simulink model "viet_HC_arbot_v2offset"  (R2020a)
settings: Solver=ode15s  StartTime=0.0  StopTime=15  MaxStep=.01  RelTol=1e-3  AbsTol=1e-4
InitFcn:
  | % currentFolder = pwd;
  | % parent = '../Targeting';
  | % environment = '../Environment';
  | % addpath(genpath(parent));
  | % addpath(genpath(environment));
  | 
  | startup_ARbot;
  | chute2_DataFile;
  | guard_DataFile1;
  | shelf_DataFile1;
  | bin_assembly_DataFile;
values from neighbouring files (symbols this model uses):
  base_link = which('base_link.STL')    [init_root_paths_mac.m]    (also in init_root_paths_windows.m)
  Environment = append(cwd,'/Environment')    [init_root_paths_mac.m]    (also in init_root_paths_windows.m = append(cwd,'\Environment'))
  L1 = which('L1.STL')    [init_root_paths_mac.m]    (also in init_root_paths_windows.m)
  L2 = which('L2.STL')    [init_root_paths_mac.m]    (also in init_root_paths_windows.m)
  L3 = which('L3.STL')    [init_root_paths_mac.m]    (also in init_root_paths_windows.m)
  L4 = which('L4.STL')    [init_root_paths_mac.m]    (also in init_root_paths_windows.m)
undefined symbols (not defined in the file or in its folder): belt_h, belt_l, belt_spd, belt_w, box1_dim, box2_dim, box3_dim, box4_dim, box5_dim, cube_d, deposit_joint_angle, Extr_Data_LinkHoles, floor_d, floor_l, ikSol, initial_joints, m, n, P_C, safe_via_angles, sigbuilder_block, smiData, X, Y, Z
libraries: sm_lib x145, nesl_utility x78, Contact_Forces_Lib x10, simulink x5, Parts_Lib x5, dspsrcs4 x1
(part 5 of 5)

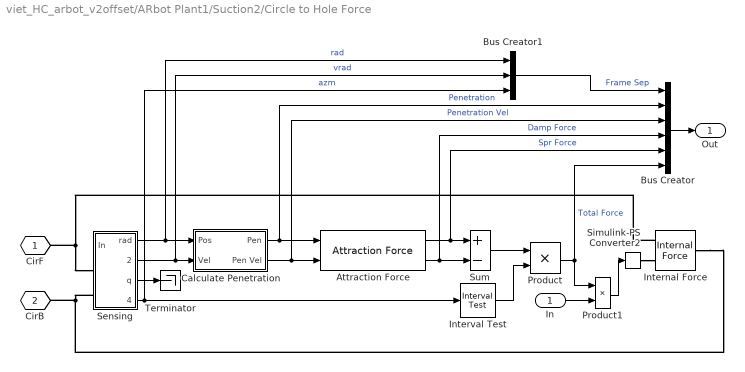
== system viet_HC_arbot_v2offset/ARbot Plant1/Suction2/Circle to Hole Force ==
  In : Inport
  Attraction Force : Contact_Forces_Lib/Other Forces/Attraction Force  k_pen=k_contact  b_penvel=b_contact  max_sep=max_frame_sep  deadzone=h_deadzone
      settings: SourceProductName=Simscape Multibody Contact Forces Library
  Bus Creator : BusCreator  Inputs=6
  Bus Creator1 : BusCreator  Inputs=3
  Calculate Penetration : Subsystem
  Internal Force : sm_lib/Forces and Torques/Internal Force
      settings: SourceProductBaseCode=MS
  Interval Test : simulink/Logic and Bit Operations/Interval Test  IntervalClosedRight=on  uplimit=active_angle(2)  IntervalClosedLeft=on  lowlimit=active_angle(1)  OutDataTypeStr=uint8
  Product : Product
  Product1 : Product
  Sensing : Subsystem
  Simulink-PS Converter2 : nesl_utility/Simulink-PS Converter  PhysicalDomain=network_engine_domain  SubClassName=ps_input  LeftPortType=input  RightPortType=output  PseudoPeriodic=off  Frequencies=[]  NoiseDistribution=none  NoiseParameters=[]  Unit=1  AffineConversion=off  FilteringAndDerivatives=zero  SimscapeFilterOrder=1  InputFilterTimeConstant=0.005  UdotUserProvided=[]
  Sum : Sum  Inputs=+-
  Terminator : Terminator
  CirF : PMIOPort  Tag=PMCPort  Side=Left
  CirB : PMIOPort  Tag=PMCPort  Port=2  Side=Right
  Out : Outport  VectorParamsAs1DForOutWhenUnconnected=off
  wires:
  Product1/1 -> Simulink-PS Converter2/1
  In/1 -> Product1/2
  Interval Test/1 -> Product/2
  Sensing/3(q) -> Terminator/1
  Sum/1 -> Product/1
  Attraction Force/1 -> Bus Creator/5, Sum/1  "Spr Force"
  Sensing/1(rad) -> Bus Creator1/1, Calculate Penetration/1(Pos)  "rad"
  Attraction Force/2 -> Bus Creator/4, Sum/2  "Damp Force"
  Sensing/2(vrad) -> Bus Creator1/2, Calculate Penetration/2(Vel)  "vrad"
  Calculate Penetration/2(Pen Vel) -> Attraction Force/2, Bus Creator/3  "Penetration Vel"
  Product/1 -> Bus Creator/6, Product1/1  "Total Force"
  Sensing/4(azm) -> Bus Creator1/3, Interval Test/1  "azm"
  Bus Creator1/1 -> Bus Creator/1  "Frame Sep"
  Calculate Penetration/1(Pen) -> Attraction Force/1, Bus Creator/2  "Penetration"
  Bus Creator/1 -> Out/1
  connections:
  Sensing/LConn2 -- Internal Force/RConn1 -- CirB/RConn1
  Internal Force/LConn1 -- Sensing/LConn1 -- CirF/RConn1
  Simulink-PS Converter2/RConn1 -- Internal Force/LConn2

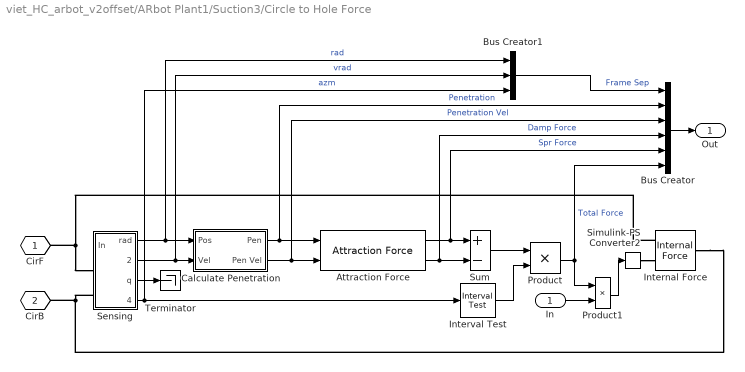
== system viet_HC_arbot_v2offset/ARbot Plant1/Suction3/Circle to Hole Force ==
  In : Inport
  Attraction Force : Contact_Forces_Lib/Other Forces/Attraction Force  k_pen=k_contact  b_penvel=b_contact  max_sep=max_frame_sep  deadzone=h_deadzone
      settings: SourceProductName=Simscape Multibody Contact Forces Library
  Bus Creator : BusCreator  Inputs=6
  Bus Creator1 : BusCreator  Inputs=3
  Calculate Penetration : Subsystem
  Internal Force : sm_lib/Forces and Torques/Internal Force
      settings: SourceProductBaseCode=MS
  Interval Test : simulink/Logic and Bit Operations/Interval Test  IntervalClosedRight=on  uplimit=active_angle(2)  IntervalClosedLeft=on  lowlimit=active_angle(1)  OutDataTypeStr=uint8
  Product : Product
  Product1 : Product
  Sensing : Subsystem
  Simulink-PS Converter2 : nesl_utility/Simulink-PS Converter  PhysicalDomain=network_engine_domain  SubClassName=ps_input  LeftPortType=input  RightPortType=output  PseudoPeriodic=off  Frequencies=[]  NoiseDistribution=none  NoiseParameters=[]  Unit=1  AffineConversion=off  FilteringAndDerivatives=zero  SimscapeFilterOrder=1  InputFilterTimeConstant=0.005  UdotUserProvided=[]
  Sum : Sum  Inputs=+-
  Terminator : Terminator
  CirF : PMIOPort  Tag=PMCPort  Side=Left
  CirB : PMIOPort  Tag=PMCPort  Port=2  Side=Right
  Out : Outport  VectorParamsAs1DForOutWhenUnconnected=off
  wires:
  Bus Creator/1 -> Out/1
  Calculate Penetration/1(Pen) -> Bus Creator/2, Attraction Force/1  "Penetration"
  Bus Creator1/1 -> Bus Creator/1  "Frame Sep"
  Sensing/4(azm) -> Interval Test/1, Bus Creator1/3  "azm"
  Product/1 -> Product1/1, Bus Creator/6  "Total Force"
  Calculate Penetration/2(Pen Vel) -> Bus Creator/3, Attraction Force/2  "Penetration Vel"
  Sensing/2(vrad) -> Calculate Penetration/2(Vel), Bus Creator1/2  "vrad"
  Attraction Force/2 -> Sum/2, Bus Creator/4  "Damp Force"
  Sensing/1(rad) -> Calculate Penetration/1(Pos), Bus Creator1/1  "rad"
  Attraction Force/1 -> Sum/1, Bus Creator/5  "Spr Force"
  Sum/1 -> Product/1
  Sensing/3(q) -> Terminator/1
  Interval Test/1 -> Product/2
  In/1 -> Product1/2
  Product1/1 -> Simulink-PS Converter2/1
  connections:
  Simulink-PS Converter2/RConn1 -- Internal Force/LConn2
  CirF/RConn1 -- Sensing/LConn1 -- Internal Force/LConn1
  CirB/RConn1 -- Internal Force/RConn1 -- Sensing/LConn2

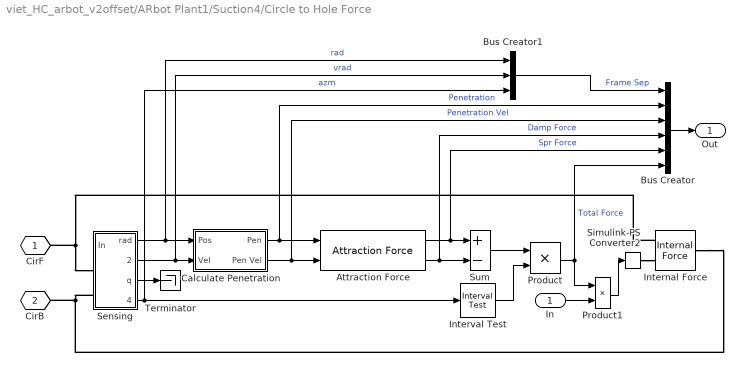
== system viet_HC_arbot_v2offset/ARbot Plant1/Suction4/Circle to Hole Force ==
  In : Inport
  Attraction Force : Contact_Forces_Lib/Other Forces/Attraction Force  k_pen=k_contact  b_penvel=b_contact  max_sep=max_frame_sep  deadzone=h_deadzone
      settings: SourceProductName=Simscape Multibody Contact Forces Library
  Bus Creator : BusCreator  Inputs=6
  Bus Creator1 : BusCreator  Inputs=3
  Calculate Penetration : Subsystem
  Internal Force : sm_lib/Forces and Torques/Internal Force
      settings: SourceProductBaseCode=MS
  Interval Test : simulink/Logic and Bit Operations/Interval Test  IntervalClosedRight=on  uplimit=active_angle(2)  IntervalClosedLeft=on  lowlimit=active_angle(1)  OutDataTypeStr=uint8
  Product : Product
  Product1 : Product
  Sensing : Subsystem
  Simulink-PS Converter2 : nesl_utility/Simulink-PS Converter  PhysicalDomain=network_engine_domain  SubClassName=ps_input  LeftPortType=input  RightPortType=output  PseudoPeriodic=off  Frequencies=[]  NoiseDistribution=none  NoiseParameters=[]  Unit=1  AffineConversion=off  FilteringAndDerivatives=zero  SimscapeFilterOrder=1  InputFilterTimeConstant=0.005  UdotUserProvided=[]
  Sum : Sum  Inputs=+-
  Terminator : Terminator
  CirF : PMIOPort  Tag=PMCPort  Side=Left
  CirB : PMIOPort  Tag=PMCPort  Port=2  Side=Right
  Out : Outport  VectorParamsAs1DForOutWhenUnconnected=off
  wires:
  Product1/1 -> Simulink-PS Converter2/1
  In/1 -> Product1/2
  Interval Test/1 -> Product/2
  Sensing/3(q) -> Terminator/1
  Sum/1 -> Product/1
  Attraction Force/1 -> Bus Creator/5, Sum/1  "Spr Force"
  Sensing/1(rad) -> Bus Creator1/1, Calculate Penetration/1(Pos)  "rad"
  Attraction Force/2 -> Bus Creator/4, Sum/2  "Damp Force"
  Sensing/2(vrad) -> Bus Creator1/2, Calculate Penetration/2(Vel)  "vrad"
  Calculate Penetration/2(Pen Vel) -> Attraction Force/2, Bus Creator/3  "Penetration Vel"
  Product/1 -> Bus Creator/6, Product1/1  "Total Force"
  Sensing/4(azm) -> Bus Creator1/3, Interval Test/1  "azm"
  Bus Creator1/1 -> Bus Creator/1  "Frame Sep"
  Calculate Penetration/1(Pen) -> Attraction Force/1, Bus Creator/2  "Penetration"
  Bus Creator/1 -> Out/1
  connections:
  Sensing/LConn2 -- Internal Force/RConn1 -- CirB/RConn1
  Internal Force/LConn1 -- Sensing/LConn1 -- CirF/RConn1
  Simulink-PS Converter2/RConn1 -- Internal Force/LConn2

== system viet_HC_arbot_v2offset/ARbot Plant1/Suction5/Circle to Hole Force ==
  In : Inport
  Attraction Force : Contact_Forces_Lib/Other Forces/Attraction Force  k_pen=k_contact  b_penvel=b_contact  max_sep=max_frame_sep  deadzone=h_deadzone
      settings: SourceProductName=Simscape Multibody Contact Forces Library
  Bus Creator : BusCreator  Inputs=6
  Bus Creator1 : BusCreator  Inputs=3
  Calculate Penetration : Subsystem
  Internal Force : sm_lib/Forces and Torques/Internal Force
      settings: SourceProductBaseCode=MS
  Interval Test : simulink/Logic and Bit Operations/Interval Test  IntervalClosedRight=on  uplimit=active_angle(2)  IntervalClosedLeft=on  lowlimit=active_angle(1)  OutDataTypeStr=uint8
  Product : Product
  Product1 : Product
  Sensing : Subsystem
  Simulink-PS Converter2 : nesl_utility/Simulink-PS Converter  PhysicalDomain=network_engine_domain  SubClassName=ps_input  LeftPortType=input  RightPortType=output  PseudoPeriodic=off  Frequencies=[]  NoiseDistribution=none  NoiseParameters=[]  Unit=1  AffineConversion=off  FilteringAndDerivatives=zero  SimscapeFilterOrder=1  InputFilterTimeConstant=0.005  UdotUserProvided=[]
  Sum : Sum  Inputs=+-
  Terminator : Terminator
  CirF : PMIOPort  Tag=PMCPort  Side=Left
  CirB : PMIOPort  Tag=PMCPort  Port=2  Side=Right
  Out : Outport  VectorParamsAs1DForOutWhenUnconnected=off
  wires:
  Bus Creator/1 -> Out/1
  Calculate Penetration/1(Pen) -> Bus Creator/2, Attraction Force/1  "Penetration"
  Bus Creator1/1 -> Bus Creator/1  "Frame Sep"
  Sensing/4(azm) -> Interval Test/1, Bus Creator1/3  "azm"
  Product/1 -> Product1/1, Bus Creator/6  "Total Force"
  Calculate Penetration/2(Pen Vel) -> Bus Creator/3, Attraction Force/2  "Penetration Vel"
  Sensing/2(vrad) -> Calculate Penetration/2(Vel), Bus Creator1/2  "vrad"
  Attraction Force/2 -> Sum/2, Bus Creator/4  "Damp Force"
  Sensing/1(rad) -> Calculate Penetration/1(Pos), Bus Creator1/1  "rad"
  Attraction Force/1 -> Sum/1, Bus Creator/5  "Spr Force"
  Sum/1 -> Product/1
  Sensing/3(q) -> Terminator/1
  Interval Test/1 -> Product/2
  In/1 -> Product1/2
  Product1/1 -> Simulink-PS Converter2/1
  connections:
  Simulink-PS Converter2/RConn1 -- Internal Force/LConn2
  CirF/RConn1 -- Sensing/LConn1 -- Internal Force/LConn1
  CirB/RConn1 -- Internal Force/RConn1 -- Sensing/LConn2

== system viet_HC_arbot_v2offset/ARbot Plant1/Suction1/Circle to Hole Force/Calculate Penetration ==
  Pos : Inport
  Vel : Inport  Port=2
  Constant : Constant  Value=max_frame_sep
  Dead Zone Outside : DeadZone  LowerValue=-inf  UpperValue=0  SaturateOnIntegerOverflow=on
  Gain2 : Gain  Gain=-1
  Sum1 : Sum  Inputs=|-+
  Pen : Outport  VectorParamsAs1DForOutWhenUnconnected=off
  Pen Vel : Outport  Port=2  VectorParamsAs1DForOutWhenUnconnected=off
  wires:
  Vel/1 -> Gain2/1
  Gain2/1 -> Pen Vel/1
  Dead Zone Outside/1 -> Pen/1
  Constant/1 -> Sum1/2
  Sum1/1 -> Dead Zone Outside/1
  Pos/1 -> Sum1/1

== system viet_HC_arbot_v2offset/ARbot Plant1/Suction1/Circle to Hole Force/Sensing ==
  In : Inport
  PS-Simulink Converter1 : nesl_utility/PS-Simulink Converter  PhysicalDomain=network_engine_domain  SubClassName=ps_output  LeftPortType=input  RightPortType=output  PseudoPeriodic=off  Frequencies=[]  Unit=deg  AffineConversion=off
  PS-Simulink Converter4 : nesl_utility/PS-Simulink Converter  PhysicalDomain=network_engine_domain  SubClassName=ps_output  LeftPortType=input  RightPortType=output  PseudoPeriodic=off  Frequencies=[]  Unit=1  AffineConversion=off
  PS-Simulink Converter5 : nesl_utility/PS-Simulink Converter  PhysicalDomain=network_engine_domain  SubClassName=ps_output  LeftPortType=input  RightPortType=output  PseudoPeriodic=off  Frequencies=[]  Unit=1  AffineConversion=off
  PS-Simulink Converter6 : nesl_utility/PS-Simulink Converter  PhysicalDomain=network_engine_domain  SubClassName=ps_output  LeftPortType=input  RightPortType=output  PseudoPeriodic=off  Frequencies=[]  Unit=1  AffineConversion=off
  Product : Product
  Selector : Selector  NumberOfDimensions=2  InputPortWidth=3  IndexOptions=Index vector (dialog),Index vector (dialog)  Indices=[1],[1,2]  OutputSizes=1,1
  Sign : Signum  ZeroCross=off
  Transform Sensor : sm_lib/Frames and Transforms/Transform Sensor  MeasurementFrame=NonRotatingBase  SenseAngle=off  SenseAxis=off  SenseAngle1=off  SenseAngle2=off  SenseAngle3=off  SenseQ=off  SenseR=off  SenseOmegaX=off  SenseOmegaY=off  SenseOmegaZ=off  SenseOmega1=off  SenseOmega2=off  SenseOmega3=off  SenseQDot=off  SenseRDot=off  SenseAlphaX=off  SenseAlphaY=off  SenseAlphaZ=off  SenseAlpha1=off  SenseAlpha2=off  SenseAlpha3=off  SenseQDDot=off  SenseRDDot=off  SenseX=off  SenseY=off  SenseZ=off  SenseRad=on  SenseAzim=on  SenseDist=off  SenseInc=off  SenseXDot=off  SenseYDot=off  SenseZDot=off  SenseRadDot=on  SenseAzimDot=off  SenseDistDot=off  SenseIncDot=off  SenseXDDot=off  SenseYDDot=off  SenseZDDot=off  SenseRadDDot=off  SenseAzimDDot=off  SenseDistDDot=off  SenseIncDDot=off
  Transform Sensor1 : sm_lib/Frames and Transforms/Transform Sensor  MeasurementFrame=World  SenseAngle=off  SenseAxis=off  SenseAngle1=off  SenseAngle2=off  SenseAngle3=off  SenseQ=off  SenseR=on  SenseOmegaX=off  SenseOmegaY=off  SenseOmegaZ=off  SenseOmega1=off  SenseOmega2=off  SenseOmega3=off  SenseQDot=off  SenseRDot=off  SenseAlphaX=off  SenseAlphaY=off  SenseAlphaZ=off  SenseAlpha1=off  SenseAlpha2=off  SenseAlpha3=off  SenseQDDot=off  SenseRDDot=off  SenseX=off  SenseY=off  SenseZ=off  SenseRad=off  SenseAzim=off  SenseDist=off  SenseInc=off  SenseXDot=off  SenseYDot=off  SenseZDot=off  SenseRadDot=off  SenseAzimDot=off  SenseDistDot=off  SenseIncDot=off  SenseXDDot=off  SenseYDDot=off  SenseZDDot=off  SenseRadDDot=off  SenseAzimDDot=off  SenseDistDDot=off  SenseIncDDot=off
  F : PMIOPort  Side=Left
  B : PMIOPort  Port=2  Side=Left
  rad : Outport  VectorParamsAs1DForOutWhenUnconnected=off
  vrad : Outport  Port=2  VectorParamsAs1DForOutWhenUnconnected=off
  q : Outport  Port=3  VectorParamsAs1DForOutWhenUnconnected=off
  azm : Outport  Port=4  VectorParamsAs1DForOutWhenUnconnected=off
  wires:
  PS-Simulink Converter6/1 -> Selector/1
  Selector/1 -> q/1
  PS-Simulink Converter1/1 -> azm/1
  PS-Simulink Converter5/1 -> Sign/1, rad/1
  In/1 -> Product/2
  Product/1 -> ?
  Sign/1 -> Product/1
  PS-Simulink Converter4/1 -> vrad/1
  connections:
  F/RConn1 -- Transform Sensor/RConn1 -- Transform Sensor1/RConn1
  Transform Sensor/LConn1 -- B/RConn1 -- Transform Sensor1/LConn1
  PS-Simulink Converter6/LConn1 -- Transform Sensor1/RConn2
  PS-Simulink Converter1/LConn1 -- Transform Sensor/RConn3
  PS-Simulink Converter5/LConn1 -- Transform Sensor/RConn2
  PS-Simulink Converter4/LConn1 -- Transform Sensor/RConn4

== system viet_HC_arbot_v2offset/ARbot Plant1/Suction2/Circle to Hole Force/Calculate Penetration ==
  Pos : Inport
  Vel : Inport  Port=2
  Constant : Constant  Value=max_frame_sep
  Dead Zone Outside : DeadZone  LowerValue=-inf  UpperValue=0  SaturateOnIntegerOverflow=on
  Gain2 : Gain  Gain=-1
  Sum1 : Sum  Inputs=|-+
  Pen : Outport  VectorParamsAs1DForOutWhenUnconnected=off
  Pen Vel : Outport  Port=2  VectorParamsAs1DForOutWhenUnconnected=off
  wires:
  Pos/1 -> Sum1/1
  Sum1/1 -> Dead Zone Outside/1
  Constant/1 -> Sum1/2
  Dead Zone Outside/1 -> Pen/1
  Gain2/1 -> Pen Vel/1
  Vel/1 -> Gain2/1

== system viet_HC_arbot_v2offset/ARbot Plant1/Suction2/Circle to Hole Force/Sensing ==
  In : Inport
  PS-Simulink Converter1 : nesl_utility/PS-Simulink Converter  PhysicalDomain=network_engine_domain  SubClassName=ps_output  LeftPortType=input  RightPortType=output  PseudoPeriodic=off  Frequencies=[]  Unit=deg  AffineConversion=off
  PS-Simulink Converter4 : nesl_utility/PS-Simulink Converter  PhysicalDomain=network_engine_domain  SubClassName=ps_output  LeftPortType=input  RightPortType=output  PseudoPeriodic=off  Frequencies=[]  Unit=1  AffineConversion=off
  PS-Simulink Converter5 : nesl_utility/PS-Simulink Converter  PhysicalDomain=network_engine_domain  SubClassName=ps_output  LeftPortType=input  RightPortType=output  PseudoPeriodic=off  Frequencies=[]  Unit=1  AffineConversion=off
  PS-Simulink Converter6 : nesl_utility/PS-Simulink Converter  PhysicalDomain=network_engine_domain  SubClassName=ps_output  LeftPortType=input  RightPortType=output  PseudoPeriodic=off  Frequencies=[]  Unit=1  AffineConversion=off
  Product : Product
  Selector : Selector  NumberOfDimensions=2  InputPortWidth=3  IndexOptions=Index vector (dialog),Index vector (dialog)  Indices=[1],[1,2]  OutputSizes=1,1
  Sign : Signum  ZeroCross=off
  Transform Sensor : sm_lib/Frames and Transforms/Transform Sensor  MeasurementFrame=NonRotatingBase  SenseAngle=off  SenseAxis=off  SenseAngle1=off  SenseAngle2=off  SenseAngle3=off  SenseQ=off  SenseR=off  SenseOmegaX=off  SenseOmegaY=off  SenseOmegaZ=off  SenseOmega1=off  SenseOmega2=off  SenseOmega3=off  SenseQDot=off  SenseRDot=off  SenseAlphaX=off  SenseAlphaY=off  SenseAlphaZ=off  SenseAlpha1=off  SenseAlpha2=off  SenseAlpha3=off  SenseQDDot=off  SenseRDDot=off  SenseX=off  SenseY=off  SenseZ=off  SenseRad=on  SenseAzim=on  SenseDist=off  SenseInc=off  SenseXDot=off  SenseYDot=off  SenseZDot=off  SenseRadDot=on  SenseAzimDot=off  SenseDistDot=off  SenseIncDot=off  SenseXDDot=off  SenseYDDot=off  SenseZDDot=off  SenseRadDDot=off  SenseAzimDDot=off  SenseDistDDot=off  SenseIncDDot=off
  Transform Sensor1 : sm_lib/Frames and Transforms/Transform Sensor  MeasurementFrame=World  SenseAngle=off  SenseAxis=off  SenseAngle1=off  SenseAngle2=off  SenseAngle3=off  SenseQ=off  SenseR=on  SenseOmegaX=off  SenseOmegaY=off  SenseOmegaZ=off  SenseOmega1=off  SenseOmega2=off  SenseOmega3=off  SenseQDot=off  SenseRDot=off  SenseAlphaX=off  SenseAlphaY=off  SenseAlphaZ=off  SenseAlpha1=off  SenseAlpha2=off  SenseAlpha3=off  SenseQDDot=off  SenseRDDot=off  SenseX=off  SenseY=off  SenseZ=off  SenseRad=off  SenseAzim=off  SenseDist=off  SenseInc=off  SenseXDot=off  SenseYDot=off  SenseZDot=off  SenseRadDot=off  SenseAzimDot=off  SenseDistDot=off  SenseIncDot=off  SenseXDDot=off  SenseYDDot=off  SenseZDDot=off  SenseRadDDot=off  SenseAzimDDot=off  SenseDistDDot=off  SenseIncDDot=off
  F : PMIOPort  Side=Left
  B : PMIOPort  Port=2  Side=Left
  rad : Outport  VectorParamsAs1DForOutWhenUnconnected=off
  vrad : Outport  Port=2  VectorParamsAs1DForOutWhenUnconnected=off
  q : Outport  Port=3  VectorParamsAs1DForOutWhenUnconnected=off
  azm : Outport  Port=4  VectorParamsAs1DForOutWhenUnconnected=off
  wires:
  PS-Simulink Converter4/1 -> vrad/1
  Sign/1 -> Product/1
  Product/1 -> ?
  In/1 -> Product/2
  PS-Simulink Converter5/1 -> rad/1, Sign/1
  PS-Simulink Converter1/1 -> azm/1
  Selector/1 -> q/1
  PS-Simulink Converter6/1 -> Selector/1
  connections:
  PS-Simulink Converter4/LConn1 -- Transform Sensor/RConn4
  PS-Simulink Converter5/LConn1 -- Transform Sensor/RConn2
  PS-Simulink Converter1/LConn1 -- Transform Sensor/RConn3
  PS-Simulink Converter6/LConn1 -- Transform Sensor1/RConn2
  Transform Sensor1/LConn1 -- B/RConn1 -- Transform Sensor/LConn1
  Transform Sensor1/RConn1 -- Transform Sensor/RConn1 -- F/RConn1

== system viet_HC_arbot_v2offset/ARbot Plant1/Suction3/Circle to Hole Force/Calculate Penetration ==
  Pos : Inport
  Vel : Inport  Port=2
  Constant : Constant  Value=max_frame_sep
  Dead Zone Outside : DeadZone  LowerValue=-inf  UpperValue=0  SaturateOnIntegerOverflow=on
  Gain2 : Gain  Gain=-1
  Sum1 : Sum  Inputs=|-+
  Pen : Outport  VectorParamsAs1DForOutWhenUnconnected=off
  Pen Vel : Outport  Port=2  VectorParamsAs1DForOutWhenUnconnected=off
  wires:
  Vel/1 -> Gain2/1
  Gain2/1 -> Pen Vel/1
  Dead Zone Outside/1 -> Pen/1
  Constant/1 -> Sum1/2
  Sum1/1 -> Dead Zone Outside/1
  Pos/1 -> Sum1/1

== system viet_HC_arbot_v2offset/ARbot Plant1/Suction3/Circle to Hole Force/Sensing ==
  In : Inport
  PS-Simulink Converter1 : nesl_utility/PS-Simulink Converter  PhysicalDomain=network_engine_domain  SubClassName=ps_output  LeftPortType=input  RightPortType=output  PseudoPeriodic=off  Frequencies=[]  Unit=deg  AffineConversion=off
  PS-Simulink Converter4 : nesl_utility/PS-Simulink Converter  PhysicalDomain=network_engine_domain  SubClassName=ps_output  LeftPortType=input  RightPortType=output  PseudoPeriodic=off  Frequencies=[]  Unit=1  AffineConversion=off
  PS-Simulink Converter5 : nesl_utility/PS-Simulink Converter  PhysicalDomain=network_engine_domain  SubClassName=ps_output  LeftPortType=input  RightPortType=output  PseudoPeriodic=off  Frequencies=[]  Unit=1  AffineConversion=off
  PS-Simulink Converter6 : nesl_utility/PS-Simulink Converter  PhysicalDomain=network_engine_domain  SubClassName=ps_output  LeftPortType=input  RightPortType=output  PseudoPeriodic=off  Frequencies=[]  Unit=1  AffineConversion=off
  Product : Product
  Selector : Selector  NumberOfDimensions=2  InputPortWidth=3  IndexOptions=Index vector (dialog),Index vector (dialog)  Indices=[1],[1,2]  OutputSizes=1,1
  Sign : Signum  ZeroCross=off
  Transform Sensor : sm_lib/Frames and Transforms/Transform Sensor  MeasurementFrame=NonRotatingBase  SenseAngle=off  SenseAxis=off  SenseAngle1=off  SenseAngle2=off  SenseAngle3=off  SenseQ=off  SenseR=off  SenseOmegaX=off  SenseOmegaY=off  SenseOmegaZ=off  SenseOmega1=off  SenseOmega2=off  SenseOmega3=off  SenseQDot=off  SenseRDot=off  SenseAlphaX=off  SenseAlphaY=off  SenseAlphaZ=off  SenseAlpha1=off  SenseAlpha2=off  SenseAlpha3=off  SenseQDDot=off  SenseRDDot=off  SenseX=off  SenseY=off  SenseZ=off  SenseRad=on  SenseAzim=on  SenseDist=off  SenseInc=off  SenseXDot=off  SenseYDot=off  SenseZDot=off  SenseRadDot=on  SenseAzimDot=off  SenseDistDot=off  SenseIncDot=off  SenseXDDot=off  SenseYDDot=off  SenseZDDot=off  SenseRadDDot=off  SenseAzimDDot=off  SenseDistDDot=off  SenseIncDDot=off
  Transform Sensor1 : sm_lib/Frames and Transforms/Transform Sensor  MeasurementFrame=World  SenseAngle=off  SenseAxis=off  SenseAngle1=off  SenseAngle2=off  SenseAngle3=off  SenseQ=off  SenseR=on  SenseOmegaX=off  SenseOmegaY=off  SenseOmegaZ=off  SenseOmega1=off  SenseOmega2=off  SenseOmega3=off  SenseQDot=off  SenseRDot=off  SenseAlphaX=off  SenseAlphaY=off  SenseAlphaZ=off  SenseAlpha1=off  SenseAlpha2=off  SenseAlpha3=off  SenseQDDot=off  SenseRDDot=off  SenseX=off  SenseY=off  SenseZ=off  SenseRad=off  SenseAzim=off  SenseDist=off  SenseInc=off  SenseXDot=off  SenseYDot=off  SenseZDot=off  SenseRadDot=off  SenseAzimDot=off  SenseDistDot=off  SenseIncDot=off  SenseXDDot=off  SenseYDDot=off  SenseZDDot=off  SenseRadDDot=off  SenseAzimDDot=off  SenseDistDDot=off  SenseIncDDot=off
  F : PMIOPort  Side=Left
  B : PMIOPort  Port=2  Side=Left
  rad : Outport  VectorParamsAs1DForOutWhenUnconnected=off
  vrad : Outport  Port=2  VectorParamsAs1DForOutWhenUnconnected=off
  q : Outport  Port=3  VectorParamsAs1DForOutWhenUnconnected=off
  azm : Outport  Port=4  VectorParamsAs1DForOutWhenUnconnected=off
  wires:
  PS-Simulink Converter6/1 -> Selector/1
  Selector/1 -> q/1
  PS-Simulink Converter1/1 -> azm/1
  PS-Simulink Converter5/1 -> Sign/1, rad/1
  In/1 -> Product/2
  Product/1 -> ?
  Sign/1 -> Product/1
  PS-Simulink Converter4/1 -> vrad/1
  connections:
  F/RConn1 -- Transform Sensor/RConn1 -- Transform Sensor1/RConn1
  Transform Sensor/LConn1 -- B/RConn1 -- Transform Sensor1/LConn1
  PS-Simulink Converter6/LConn1 -- Transform Sensor1/RConn2
  PS-Simulink Converter1/LConn1 -- Transform Sensor/RConn3
  PS-Simulink Converter5/LConn1 -- Transform Sensor/RConn2
  PS-Simulink Converter4/LConn1 -- Transform Sensor/RConn4

== system viet_HC_arbot_v2offset/ARbot Plant1/Suction4/Circle to Hole Force/Calculate Penetration ==
  Pos : Inport
  Vel : Inport  Port=2
  Constant : Constant  Value=max_frame_sep
  Dead Zone Outside : DeadZone  LowerValue=-inf  UpperValue=0  SaturateOnIntegerOverflow=on
  Gain2 : Gain  Gain=-1
  Sum1 : Sum  Inputs=|-+
  Pen : Outport  VectorParamsAs1DForOutWhenUnconnected=off
  Pen Vel : Outport  Port=2  VectorParamsAs1DForOutWhenUnconnected=off
  wires:
  Pos/1 -> Sum1/1
  Sum1/1 -> Dead Zone Outside/1
  Constant/1 -> Sum1/2
  Dead Zone Outside/1 -> Pen/1
  Gain2/1 -> Pen Vel/1
  Vel/1 -> Gain2/1

== system viet_HC_arbot_v2offset/ARbot Plant1/Suction4/Circle to Hole Force/Sensing ==
  In : Inport
  PS-Simulink Converter1 : nesl_utility/PS-Simulink Converter  PhysicalDomain=network_engine_domain  SubClassName=ps_output  LeftPortType=input  RightPortType=output  PseudoPeriodic=off  Frequencies=[]  Unit=deg  AffineConversion=off
  PS-Simulink Converter4 : nesl_utility/PS-Simulink Converter  PhysicalDomain=network_engine_domain  SubClassName=ps_output  LeftPortType=input  RightPortType=output  PseudoPeriodic=off  Frequencies=[]  Unit=1  AffineConversion=off
  PS-Simulink Converter5 : nesl_utility/PS-Simulink Converter  PhysicalDomain=network_engine_domain  SubClassName=ps_output  LeftPortType=input  RightPortType=output  PseudoPeriodic=off  Frequencies=[]  Unit=1  AffineConversion=off
  PS-Simulink Converter6 : nesl_utility/PS-Simulink Converter  PhysicalDomain=network_engine_domain  SubClassName=ps_output  LeftPortType=input  RightPortType=output  PseudoPeriodic=off  Frequencies=[]  Unit=1  AffineConversion=off
  Product : Product
  Selector : Selector  NumberOfDimensions=2  InputPortWidth=3  IndexOptions=Index vector (dialog),Index vector (dialog)  Indices=[1],[1,2]  OutputSizes=1,1
  Sign : Signum  ZeroCross=off
  Transform Sensor : sm_lib/Frames and Transforms/Transform Sensor  MeasurementFrame=NonRotatingBase  SenseAngle=off  SenseAxis=off  SenseAngle1=off  SenseAngle2=off  SenseAngle3=off  SenseQ=off  SenseR=off  SenseOmegaX=off  SenseOmegaY=off  SenseOmegaZ=off  SenseOmega1=off  SenseOmega2=off  SenseOmega3=off  SenseQDot=off  SenseRDot=off  SenseAlphaX=off  SenseAlphaY=off  SenseAlphaZ=off  SenseAlpha1=off  SenseAlpha2=off  SenseAlpha3=off  SenseQDDot=off  SenseRDDot=off  SenseX=off  SenseY=off  SenseZ=off  SenseRad=on  SenseAzim=on  SenseDist=off  SenseInc=off  SenseXDot=off  SenseYDot=off  SenseZDot=off  SenseRadDot=on  SenseAzimDot=off  SenseDistDot=off  SenseIncDot=off  SenseXDDot=off  SenseYDDot=off  SenseZDDot=off  SenseRadDDot=off  SenseAzimDDot=off  SenseDistDDot=off  SenseIncDDot=off
  Transform Sensor1 : sm_lib/Frames and Transforms/Transform Sensor  MeasurementFrame=World  SenseAngle=off  SenseAxis=off  SenseAngle1=off  SenseAngle2=off  SenseAngle3=off  SenseQ=off  SenseR=on  SenseOmegaX=off  SenseOmegaY=off  SenseOmegaZ=off  SenseOmega1=off  SenseOmega2=off  SenseOmega3=off  SenseQDot=off  SenseRDot=off  SenseAlphaX=off  SenseAlphaY=off  SenseAlphaZ=off  SenseAlpha1=off  SenseAlpha2=off  SenseAlpha3=off  SenseQDDot=off  SenseRDDot=off  SenseX=off  SenseY=off  SenseZ=off  SenseRad=off  SenseAzim=off  SenseDist=off  SenseInc=off  SenseXDot=off  SenseYDot=off  SenseZDot=off  SenseRadDot=off  SenseAzimDot=off  SenseDistDot=off  SenseIncDot=off  SenseXDDot=off  SenseYDDot=off  SenseZDDot=off  SenseRadDDot=off  SenseAzimDDot=off  SenseDistDDot=off  SenseIncDDot=off
  F : PMIOPort  Side=Left
  B : PMIOPort  Port=2  Side=Left
  rad : Outport  VectorParamsAs1DForOutWhenUnconnected=off
  vrad : Outport  Port=2  VectorParamsAs1DForOutWhenUnconnected=off
  q : Outport  Port=3  VectorParamsAs1DForOutWhenUnconnected=off
  azm : Outport  Port=4  VectorParamsAs1DForOutWhenUnconnected=off
  wires:
  PS-Simulink Converter4/1 -> vrad/1
  Sign/1 -> Product/1
  Product/1 -> ?
  In/1 -> Product/2
  PS-Simulink Converter5/1 -> rad/1, Sign/1
  PS-Simulink Converter1/1 -> azm/1
  Selector/1 -> q/1
  PS-Simulink Converter6/1 -> Selector/1
  connections:
  PS-Simulink Converter4/LConn1 -- Transform Sensor/RConn4
  PS-Simulink Converter5/LConn1 -- Transform Sensor/RConn2
  PS-Simulink Converter1/LConn1 -- Transform Sensor/RConn3
  PS-Simulink Converter6/LConn1 -- Transform Sensor1/RConn2
  Transform Sensor1/LConn1 -- B/RConn1 -- Transform Sensor/LConn1
  Transform Sensor1/RConn1 -- Transform Sensor/RConn1 -- F/RConn1

== system viet_HC_arbot_v2offset/ARbot Plant1/Suction5/Circle to Hole Force/Calculate Penetration ==
  Pos : Inport
  Vel : Inport  Port=2
  Constant : Constant  Value=max_frame_sep
  Dead Zone Outside : DeadZone  LowerValue=-inf  UpperValue=0  SaturateOnIntegerOverflow=on
  Gain2 : Gain  Gain=-1
  Sum1 : Sum  Inputs=|-+
  Pen : Outport  VectorParamsAs1DForOutWhenUnconnected=off
  Pen Vel : Outport  Port=2  VectorParamsAs1DForOutWhenUnconnected=off
  wires:
  Vel/1 -> Gain2/1
  Gain2/1 -> Pen Vel/1
  Dead Zone Outside/1 -> Pen/1
  Constant/1 -> Sum1/2
  Sum1/1 -> Dead Zone Outside/1
  Pos/1 -> Sum1/1

== system viet_HC_arbot_v2offset/ARbot Plant1/Suction5/Circle to Hole Force/Sensing ==
  In : Inport
  PS-Simulink Converter1 : nesl_utility/PS-Simulink Converter  PhysicalDomain=network_engine_domain  SubClassName=ps_output  LeftPortType=input  RightPortType=output  PseudoPeriodic=off  Frequencies=[]  Unit=deg  AffineConversion=off
  PS-Simulink Converter4 : nesl_utility/PS-Simulink Converter  PhysicalDomain=network_engine_domain  SubClassName=ps_output  LeftPortType=input  RightPortType=output  PseudoPeriodic=off  Frequencies=[]  Unit=1  AffineConversion=off
  PS-Simulink Converter5 : nesl_utility/PS-Simulink Converter  PhysicalDomain=network_engine_domain  SubClassName=ps_output  LeftPortType=input  RightPortType=output  PseudoPeriodic=off  Frequencies=[]  Unit=1  AffineConversion=off
  PS-Simulink Converter6 : nesl_utility/PS-Simulink Converter  PhysicalDomain=network_engine_domain  SubClassName=ps_output  LeftPortType=input  RightPortType=output  PseudoPeriodic=off  Frequencies=[]  Unit=1  AffineConversion=off
  Product : Product
  Selector : Selector  NumberOfDimensions=2  InputPortWidth=3  IndexOptions=Index vector (dialog),Index vector (dialog)  Indices=[1],[1,2]  OutputSizes=1,1
  Sign : Signum  ZeroCross=off
  Transform Sensor : sm_lib/Frames and Transforms/Transform Sensor  MeasurementFrame=NonRotatingBase  SenseAngle=off  SenseAxis=off  SenseAngle1=off  SenseAngle2=off  SenseAngle3=off  SenseQ=off  SenseR=off  SenseOmegaX=off  SenseOmegaY=off  SenseOmegaZ=off  SenseOmega1=off  SenseOmega2=off  SenseOmega3=off  SenseQDot=off  SenseRDot=off  SenseAlphaX=off  SenseAlphaY=off  SenseAlphaZ=off  SenseAlpha1=off  SenseAlpha2=off  SenseAlpha3=off  SenseQDDot=off  SenseRDDot=off  SenseX=off  SenseY=off  SenseZ=off  SenseRad=on  SenseAzim=on  SenseDist=off  SenseInc=off  SenseXDot=off  SenseYDot=off  SenseZDot=off  SenseRadDot=on  SenseAzimDot=off  SenseDistDot=off  SenseIncDot=off  SenseXDDot=off  SenseYDDot=off  SenseZDDot=off  SenseRadDDot=off  SenseAzimDDot=off  SenseDistDDot=off  SenseIncDDot=off
  Transform Sensor1 : sm_lib/Frames and Transforms/Transform Sensor  MeasurementFrame=World  SenseAngle=off  SenseAxis=off  SenseAngle1=off  SenseAngle2=off  SenseAngle3=off  SenseQ=off  SenseR=on  SenseOmegaX=off  SenseOmegaY=off  SenseOmegaZ=off  SenseOmega1=off  SenseOmega2=off  SenseOmega3=off  SenseQDot=off  SenseRDot=off  SenseAlphaX=off  SenseAlphaY=off  SenseAlphaZ=off  SenseAlpha1=off  SenseAlpha2=off  SenseAlpha3=off  SenseQDDot=off  SenseRDDot=off  SenseX=off  SenseY=off  SenseZ=off  SenseRad=off  SenseAzim=off  SenseDist=off  SenseInc=off  SenseXDot=off  SenseYDot=off  SenseZDot=off  SenseRadDot=off  SenseAzimDot=off  SenseDistDot=off  SenseIncDot=off  SenseXDDot=off  SenseYDDot=off  SenseZDDot=off  SenseRadDDot=off  SenseAzimDDot=off  SenseDistDDot=off  SenseIncDDot=off
  F : PMIOPort  Side=Left
  B : PMIOPort  Port=2  Side=Left
  rad : Outport  VectorParamsAs1DForOutWhenUnconnected=off
  vrad : Outport  Port=2  VectorParamsAs1DForOutWhenUnconnected=off
  q : Outport  Port=3  VectorParamsAs1DForOutWhenUnconnected=off
  azm : Outport  Port=4  VectorParamsAs1DForOutWhenUnconnected=off
  wires:
  PS-Simulink Converter6/1 -> Selector/1
  Selector/1 -> q/1
  PS-Simulink Converter1/1 -> azm/1
  PS-Simulink Converter5/1 -> Sign/1, rad/1
  In/1 -> Product/2
  Product/1 -> ?
  Sign/1 -> Product/1
  PS-Simulink Converter4/1 -> vrad/1
  connections:
  F/RConn1 -- Transform Sensor/RConn1 -- Transform Sensor1/RConn1
  Transform Sensor/LConn1 -- B/RConn1 -- Transform Sensor1/LConn1
  PS-Simulink Converter6/LConn1 -- Transform Sensor1/RConn2
  PS-Simulink Converter1/LConn1 -- Transform Sensor/RConn3
  PS-Simulink Converter5/LConn1 -- Transform Sensor/RConn2
  PS-Simulink Converter4/LConn1 -- Transform Sensor/RConn4

== stateflow chart viet_HC_arbot_v2offset/traj_receiver1 ==
  settings: updateMethod=DISCRETE  sampleTime=0.02
  state traj_inc [commented out]
    en:
    i = i + 1;
  state receive_msg
    i = 1;
    qin = initial_joints;
  state calc_Traj
    en:
    % calculate a trajectory
    q0=qin; % bin location
    qf=qin;
    th=traj6_v2(q0,safe_via_angles,ikSol(trajsExecuted,:),2,1);
    th_return=traj6_v2(ikSol(trajsExecuted,:),safe_via_angles,q0,2,1);
    th = [ th; th_return ]; % append both trajectories
    th_length = length(th); % for to target and return trajectory
  state send_Traj
    en:
    i = i + 1;
    qin = [  th(i,1)  th(i,2)  th(i,3)  th(i,4) ];
    % send(joint1Message);
  traj_inc -> receive_msg [commented out] : [i > th_length]{
      | trajsExecuted = trajsExecuted + 1}
  (default) -> receive_msg : {trajsExecuted = 1;}
  traj_inc -> send_Traj [commented out] : after(0.04,sec)
      | [i<=th_length]
  send_Traj -> traj_inc [commented out]
  send_Traj -> receive_msg [order 1] : [i >= th_length]{
      | trajsExecuted = trajsExecuted + 1}
  receive_msg -> calc_Traj : traj_Init
  calc_Traj -> send_Traj
  send_Traj -> send_Traj [order 2] : after(0.04,sec)
      | [i<th_length]
  data: traj_Init input; q0 local; qf local; th local size=[ 50 4 ]; th_length local; qin output double size=[1,4]; i local; ikSol parameter size=[5 4]; trajsExecuted local; safe_via_angles parameter size=[1 4]; th_return local; traj_receiverMode output Enum: traj_receiverModeType; initial_joints parameter size=[1 4];

== stateflow chart viet_HC_arbot_v2offset/traj_sender1 ==
  state begin_traj
    en:
    if ~isempty(ETA_array)
    if (ETA_array(1) <= 0)
    send(traj_Init);
    ETA_array(1) = [];
    end
    end
  (default) -> begin_traj : {traj_Init.data = false;
      | ETA_array = testing_array}
  begin_traj -> begin_traj : [after(100,msec)&&~isempty(ETA_array)]{ETA_array = ETA_array - 0.1;
      | }
  data: traj_Init output; ETA_array local size=[1 100]; testing_array parameter size=[1 5]
